simulink model "Single_Phase_Half_Bridge_Controlled_RL_Load"  (R2018a)
settings: Solver=VariableStepAuto  StartTime=0.0  StopTime=0.1  RelTol=1e-3
libraries: powerlib x15, powerlib_meascontrol x5
settings Model: Creator=ozie  LastModifiedBy=ozie

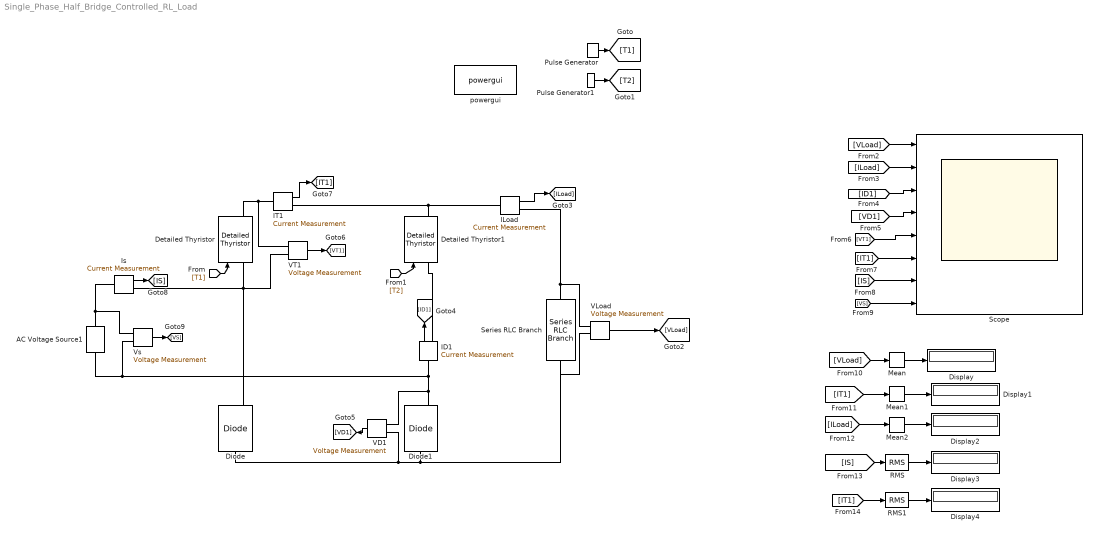
== system Single_Phase_Half_Bridge_Controlled_RL_Load ==
  " VD1" : powerlib/Measurements/Voltage Measurement  PhasorSimulation=off  OutputType=Complex  PSBequivalent=0
  " VLoad" : powerlib/Measurements/Voltage Measurement  PhasorSimulation=off  OutputType=Complex  PSBequivalent=0
  AC Voltage Source1 : powerlib/Electrical Sources/AC Voltage Source  Amplitude=220*sqrt(2)  Phase=0  Frequency=50  SampleTime=0  Measurements=None  BusType=swing  Pref=10e3  Qref=0  Qmin=-inf  Qmax=+inf
  Detailed Thyristor : powerlib/Power Electronics/Detailed Thyristor  Ron=0.001  Lon=1e-3  Vf=0.8  IL=0.1  Tq=100e-6  IC=0  Rs=500  Cs=250e-9  Measurements=on
      settings: SourceProductName=Simscape Power Systems  SourceProductBaseCode=PS
  Detailed Thyristor1 : powerlib/Power Electronics/Detailed Thyristor  Ron=0.001  Lon=1e-3  Vf=0.8  IL=0.1  Tq=100e-6  IC=0  Rs=500  Cs=250e-9  Measurements=on
      settings: SourceProductName=Simscape Power Systems  SourceProductBaseCode=PS
  Diode : powerlib/Power Electronics/Diode  Ron=0.001  Lon=0  Vf=0.8  IC=0  UseSnubber=0  Rs=500  Cs=250e-9  Measurements=on
  Diode1 : powerlib/Power Electronics/Diode  Ron=0.001  Lon=0  Vf=0.8  IC=0  UseSnubber=0  Rs=500  Cs=250e-9  Measurements=on
  Display{,1..4} (5 alike) : Display
  ID1 : powerlib/Measurements/Current Measurement  PhasorSimulation=off  OutputType=Complex  PSBequivalent=0
  ILoad : powerlib/Measurements/Current Measurement  PhasorSimulation=off  OutputType=Complex  PSBequivalent=0
  "IT1 " : powerlib/Measurements/Current Measurement  PhasorSimulation=off  OutputType=Complex  PSBequivalent=0
  Is : powerlib/Measurements/Current Measurement  PhasorSimulation=off  OutputType=Complex  PSBequivalent=0
  Mean : powerlib_meascontrol/Measurements/Mean  Freq=50  Vinit=0  Ts=0
  Mean1 : powerlib_meascontrol/Measurements/Mean  Freq=50  Vinit=0  Ts=0
  Mean2 : powerlib_meascontrol/Measurements/Mean  Freq=50  Vinit=0  Ts=0
  Pulse Generator : DiscretePulseGenerator  PulseType=Time based  Period=1/50  PulseWidth=5  PhaseDelay=(120/360)*1/50
  Pulse Generator1 : DiscretePulseGenerator  PulseType=Time based  Period=1/50  PulseWidth=5  PhaseDelay=(300/360)*1/50
  RMS : powerlib_meascontrol/Measurements/RMS  TrueRMS=on  Freq=50  RMSInit=120  Ts=0
  RMS1 : powerlib_meascontrol/Measurements/RMS  TrueRMS=on  Freq=50  RMSInit=120  Ts=0
  Scope : Scope  NumInputPorts=8
  Series RLC Branch : powerlib/Elements/Series RLC Branch  LConnTagsString=__new0  RConnTagsString=__new0  BranchType=RL  Resistance=1  Inductance=2e-3  SetiL0=off  InitialCurrent=0  Capacitance=1e-6  Setx0=off  InitialVoltage=0  Measurements=None
  "VT1 " : powerlib/Measurements/Voltage Measurement  PhasorSimulation=off  OutputType=Complex  PSBequivalent=0
  "Vs " : powerlib/Measurements/Voltage Measurement  PhasorSimulation=off  OutputType=Complex  PSBequivalent=0
  powergui : powerlib/powergui  Priority=1  SimulationMode=Continuous  SampleTime=50e-6  frequency=60  Iterations=50  frequencyindice=50  Pbase=100e6  ErrMax=1e-4  UnitsV=kV  UnitsW=MW  buscounter=0  FunctionMessages=off  echomessages=off  EnableUseOfTLC=off  CurrentSourceSwitches=off  DisableSnubberDevices=off  DisableRonSwitches=off  DisableVfSwitches=off  DisplayEquations=off  SolverType=Tustin/Backward Euler (TBE)  Interpol=off  ExternalGateDelay=off  methode=off  Ts=100  x0status=blocks  SPID=on  SwTol=0  HookPort=off  RestoreLinks=warning  ResistiveCurrentMeasurement=off  Frange=[0:2:500]  Ylog=off  Xlog=on  ShowGrid=off  save=off  variable=ZData  structure=0  ZoomFFT=off  StartTime=0.0  cycles=1  DisplayStyle=1  fundamental=60  FreqAxis=off  MaxFrequency=1000  frequencyindicesteady=1  RmsSteady=1  display=off
  wires:
  Pulse Generator/1 -> [T1]
  [T1] -> Detailed Thyristor/1
  Pulse Generator1/1 -> [T2]
  [T2] -> Detailed Thyristor1/1
  " VLoad"/1 -> [VLoad]
  [VLoad] -> Scope/1
  ILoad/1 -> [ILoad]
  [ILoad] -> Scope/2
  ID1/1 -> [ID1]
  [ID1] -> Scope/3
  " VD1"/1 -> [VD1]
  [VD1] -> Scope/4
  "VT1 "/1 -> [VT1]
  "IT1 "/1 -> [IT1]
  [VT1] -> Scope/5
  [IT1] -> Scope/6
  Is/1 -> [IS]
  "Vs "/1 -> [VS]
  [IS] -> Scope/7
  [VS] -> Scope/8
  Mean/1 -> Display/1
  [VLoad] -> Mean/1
  [IT1] -> Mean1/1
  Mean1/1 -> Display1/1
  [ILoad] -> Mean2/1
  Mean2/1 -> Display2/1
  RMS/1 -> Display3/1
  [IS] -> RMS/1
  RMS1/1 -> Display4/1
  [IT1] -> RMS1/1
  connections:
  Diode/LConn1 -- " VD1"/LConn1 -- " VLoad"/LConn2 -- Series RLC Branch/LConn1 -- Diode1/LConn1
  AC Voltage Source1/LConn1 -- ID1/LConn1 -- " VD1"/LConn2 -- Diode1/RConn1 -- "Vs "/LConn2
  Is/LConn1 -- "Vs "/LConn1 -- AC Voltage Source1/RConn1
  "IT1 "/RConn1 -- ILoad/LConn1 -- Detailed Thyristor1/RConn1
  "IT1 "/LConn1 -- "VT1 "/LConn2 -- Detailed Thyristor/RConn1
  ILoad/RConn1 -- " VLoad"/LConn1 -- Series RLC Branch/RConn1
  Detailed Thyristor/LConn1 -- "VT1 "/LConn1 -- Diode/RConn1 -- Is/RConn1
  Detailed Thyristor1/LConn1 -- ID1/RConn1
